simulink model "Pulse_Radar"  (R2026a)
settings: Solver=FixedStepDiscrete  StopTime=T_stop
values from neighbouring files (symbols this model uses):
  alpha = N_train * (Pfa^(-1/N_train) - 1)    (= 17.2776488339)    [init.m]
  cfar_delay = (N_train/2) + (N_guard/2)    (= 116)    [init.m]
  current_seed = randi(100000)    [init.m]    (also in run_monte_carlo.m)
  doppler_window = hamming(N_cpi)'    [init.m]
  drop_threshold_delay = 8    [init.m]
  fd = (2 * target_velocity) / lambda    [init.m]
  hardware_delay_samples = matched_filter_delay + cfar_delay + drop_threshold_delay    [init.m]
  lambda = c / fc    (= 0.03)    [init.m]
  MTI_delay = N_PRI    [init.m]
  N_cpi = 16    [init.m]
  N_delay = round(tau / Ts)    [init.m]
  N_PRI = round(PRI / Ts)    [init.m]
  N_tau_p = round(tau_p / Ts)    [init.m]
  noise_variance_IQ = Pn / 2    (= 3.99251989225e-15)    [init.m]
  radar_const = (Pt * G^2 * lambda^2) / (((4*pi)^3) * (R^4) * L)    [init.m]
  range_per_sample = (c * Ts) / 2    (= 150)    [init.m]
  sigma_avg = 1    [init.m]
  T_stop = N_cpi * PRI    (= 0.016)    [init.m]
  Ts = 1e-6    (= 1e-06)    [init.m]
  V_rx = sqrt(Pr)    [init.m]
undefined symbols (not defined in the file or in its folder): cfar_window, dspblkCoreblockFVToolHelper, gcbh, get, jet, magnitude, Radix
libraries: dspobslib x2, dspxfrm3 x1, simulink x1
settings Model: Creator=daksh  LastModifiedBy=daksh

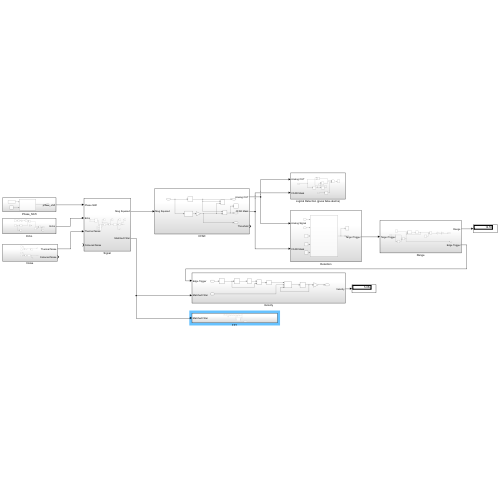
[thumbnail: Simulink's stored preview of the top-level diagram]
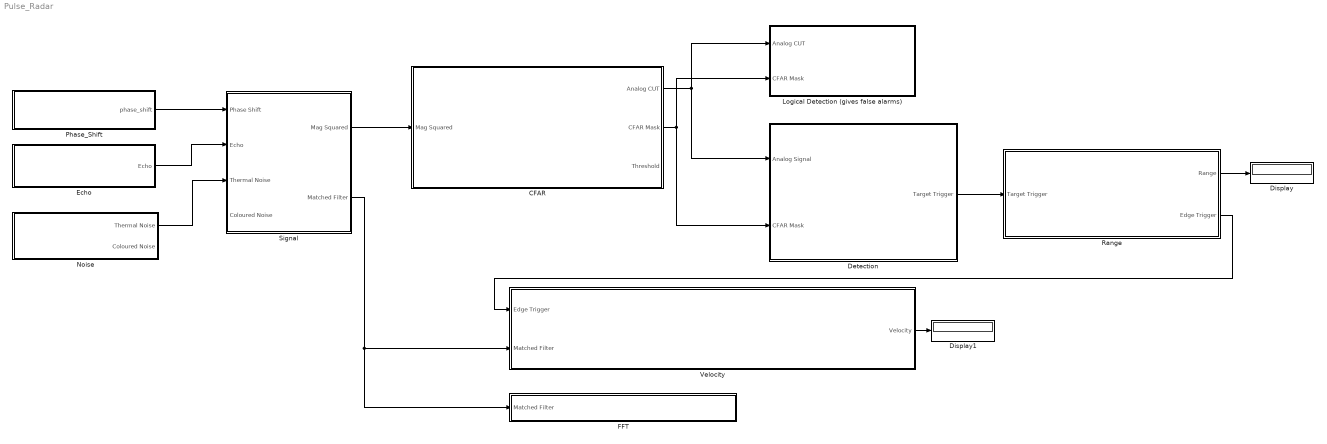
== system Pulse_Radar ==
  CFAR : Subsystem
  Detection : Subsystem
  Display : Display
  Display1 : Display
  Echo : Subsystem
  FFT : Subsystem
  Logical Detection (gives false alarms) : Subsystem
  Noise : Subsystem
  Phase_Shift : Subsystem
  Range : Subsystem
  Signal : Subsystem
  Velocity : Subsystem
  wires:
  Range/1(Range) -> Display/1
  Velocity/1(Velocity) -> Display1/1
  Echo/1(Echo) -> Signal/2(Echo)
  Noise/1(Thermal Noise) -> Signal/3(Thermal Noise)
  Signal/2(Matched Filter) -> Velocity/2(Matched Filter), FFT/1(Matched Filter)
  Signal/1(Mag Squared) -> CFAR/1(Mag Squared)
  CFAR/1(Analog CUT) -> Logical Detection (gives false alarms)/1(Analog CUT), Detection/1(Analog Signal)
  CFAR/2(CFAR Mask) -> Detection/2(CFAR Mask), Logical Detection (gives false alarms)/2(CFAR Mask)
  Detection/1(Target Trigger) -> Range/1(Target Trigger)
  Range/2(Edge Trigger) -> Velocity/1(Edge Trigger)
  Phase_Shift/1(phase_shift) -> Signal/1(Phase Shift)

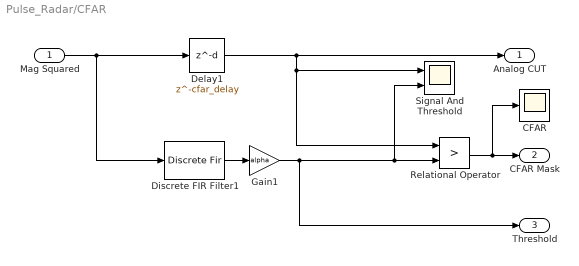
== system Pulse_Radar/CFAR ==
  Mag Squared : Inport
  CFAR : Scope
      settings: ActiveDisplayYMinimum=-0.12499999999999997  ActiveDisplayYMaximum=1.125  DataLoggingVariableName=ScopeData10
  Delay1 : Delay  DelayLength=cfar_delay
  Discrete FIR Filter1 : DiscreteFir  LoadFcn=dspblkCoreblockFVToolHelper(gcbh,'load');  Coefficients=cfar_window
      settings: CopyFcn=dspblkCoreblockFVToolHelper(gcbh,'copy');  DeleteFcn=dspblkCoreblockFVToolHelper(gcbh,'close');  ModelCloseFcn=dspblkCoreblockFVToolHelper(gcbh,'close');  PreSaveFcn=dspblkCoreblockFVToolHelper(gcbh,'presave');  PostSaveFcn=dspblkCoreblockFVToolHelper(gcbh,'postsave');  CloseFcn=dspblkCoreblockFVToolHelper(gcbh,'close');
  Gain1 : Gain  Gain=alpha
  Relational Operator : RelationalOperator  Operator=>  OutDataTypeStr=boolean  RndMeth=Simplest  InputSameDT=off
  Signal And Threshold : Scope  NumInputPorts=2
      settings: ActiveDisplayYMinimum=-1.3778826486130848E-11  ActiveDisplayYMaximum=1.2400943837517766E-10  DataLoggingVariableName=ScopeData9
  Analog CUT : Outport
  CFAR Mask : Outport  Port=2
  Threshold : Outport  Port=3
  wires:
  Gain1/1 -> Signal And Threshold/2, Relational Operator/2, Threshold/1
  Discrete FIR Filter1/1 -> Gain1/1
  Mag Squared/1 -> Discrete FIR Filter1/1, Delay1/1
  Relational Operator/1 -> CFAR/1, CFAR Mask/1
  Delay1/1 -> Relational Operator/1, Signal And Threshold/1, Analog CUT/1

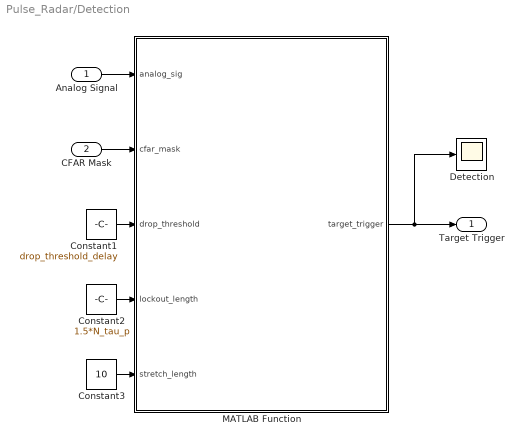
== system Pulse_Radar/Detection ==
  Analog Signal : Inport
  CFAR Mask : Inport  Port=2
  Constant1 : Constant  Value=drop_threshold_delay
  Constant2 : Constant  Value=1.5*N_tau_p
  Constant3 : Constant  Value=10
  Detection : Scope
      settings: ActiveDisplayYMinimum=-1  ActiveDisplayYMaximum=1  DataLoggingVariableName=ScopeData9
  MATLAB Function : MATLAB Function  TreatAsAtomicUnit=on
  Target Trigger : Outport
  wires:
  Constant3/1 -> MATLAB Function/5(stretch_length)
  Constant1/1 -> MATLAB Function/3(drop_threshold)
  Constant2/1 -> MATLAB Function/4(lockout_length)
  Analog Signal/1 -> MATLAB Function/1(analog_sig)
  CFAR Mask/1 -> MATLAB Function/2(cfar_mask)
  MATLAB Function/1(target_trigger) -> Detection/1, Target Trigger/1

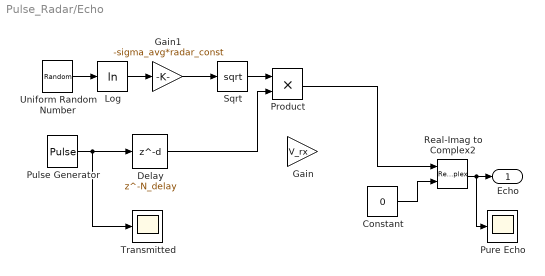
== system Pulse_Radar/Echo ==
  Constant : Constant  Value=0
  Delay : Delay  DelayLength=N_delay
  Gain : Gain  Gain=V_rx
  Gain1 : Gain  Gain=-sigma_avg*radar_const
  Log : Math  Operator=log
  Product : Product
  Pulse Generator : DiscretePulseGenerator  Period=N_PRI  PulseWidth=N_tau_p  SampleTime=Ts
  Pure Echo : Scope
      settings: ActiveDisplayYMinimum=-1.6716928323855177E-7  ActiveDisplayYMaximum=1.5045235491469661E-6  DataLoggingVariableName=ScopeData2
  Real-Imag to Complex2 : RealImagToComplex
  Sqrt : Sqrt
  Transmitted : Scope
      settings: ActiveDisplayYMinimum=-0.12499999999999997  ActiveDisplayYMaximum=1.125  DataLoggingVariableName=ScopeData3
  Uniform Random Number : UniformRandomNumber  Minimum=0.0001  Seed=current_seed  SampleTime=T_stop
  Echo : Outport
  wires:
  Pulse Generator/1 -> Transmitted/1, Delay/1
  Constant/1 -> Real-Imag to Complex2/2
  Real-Imag to Complex2/1 -> Pure Echo/1, Echo/1
  Uniform Random Number/1 -> Log/1
  Log/1 -> Gain1/1
  Gain1/1 -> Sqrt/1
  Sqrt/1 -> Product/1
  Delay/1 -> Product/2
  Product/1 -> Real-Imag to Complex2/1

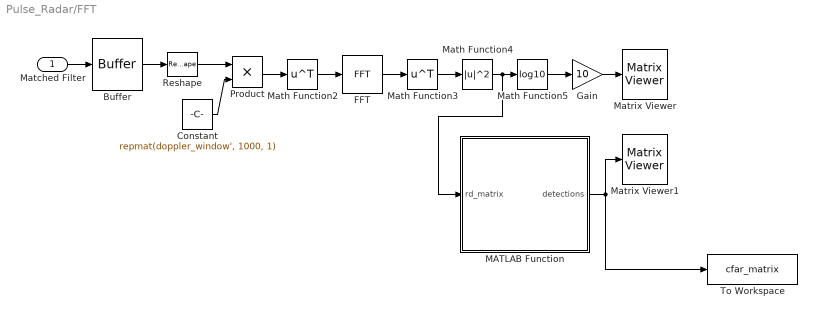
== system Pulse_Radar/FFT ==
  Matched Filter : Inport
  Buffer : Buffer  N=N_PRI*N_cpi  OutputFrames=off
  Constant : Constant  Value=repmat(doppler_window', 1000, 1)  VectorParams1D=off
  FFT : dspxfrm3/FFT  FFTImplementation=Radix-2  CompMethod=Table lookup  TableOpt=NEW  TableOptActive=Speed  BitRevOrder=off  Normalize=off  InheritFFTLength=on  FFTLength=64  WrapInput=on  roundingMode=Ceiling  overflowMode=off  firstCoeffDataTypeStr=Inherit: Same word length as input  firstCoeffLastDataTypeStr=Inherit: Same word length as input  outputMin=[]  outputMax=[]
  Gain : Gain  Gain=10
  MATLAB Function : MATLAB Function  TreatAsAtomicUnit=on
  Math Function2 : Math  Operator=transpose
  Math Function3 : Math  Operator=transpose
  Math Function4 : Math  Operator=magnitude^2
  Math Function5 : Math  Operator=log10
  Matrix Viewer : dspobslib/Matrix Viewer  ImageParams=off  CMapStr=jet(256)  AxisColorbar=on  AxisParams=off  AxisOrigin=Upper left corner  AxisTickMode=Auto  XTickRange=[0 1]  YTickRange=[0 1]  XLabel=X-axis  YLabel=Y-axis  ZLabel=Z-axis  FigPos=get(0,'defaultfigureposition')  AxisZoom=off
      settings: YMin=-100  YMax=0
  Matrix Viewer1 : dspobslib/Matrix Viewer  ImageParams=off  CMapStr=gray  AxisColorbar=on  AxisParams=off  AxisOrigin=Upper left corner  AxisTickMode=Auto  XTickRange=[0 1]  YTickRange=[0 1]  XLabel=X-axis  YLabel=Y-axis  ZLabel=Z-axis  FigPos=get(0,'defaultfigureposition')  AxisZoom=off
      settings: YMin=0  YMax=1
  Product : Product
  Reshape : Reshape  OutputDimensionality=Customize  OutputDimensions=[N_PRI, N_cpi]
  To Workspace : ToWorkspace  VariableName=cfar_matrix  SampleTime=-1
  wires:
  Math Function5/1 -> Gain/1
  Math Function3/1 -> Math Function4/1
  FFT/1 -> Math Function3/1
  Gain/1 -> Matrix Viewer/1
  Math Function4/1 -> MATLAB Function/1(rd_matrix), Math Function5/1
  Math Function2/1 -> FFT/1
  Buffer/1 -> Reshape/1
  Matched Filter/1 -> Buffer/1
  MATLAB Function/1(detections) -> Matrix Viewer1/1, To Workspace/1
  Reshape/1 -> Product/1
  Constant/1 -> Product/2
  Product/1 -> Math Function2/1

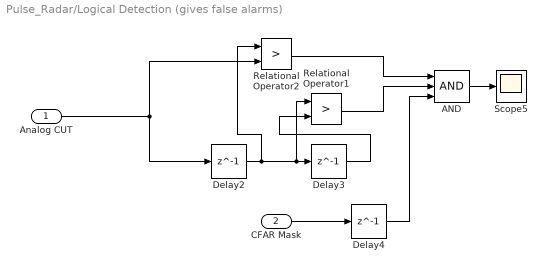
== system Pulse_Radar/Logical Detection (gives false alarms) ==
  Analog CUT : Inport
  CFAR Mask : Inport  Port=2
  AND : Logic  Inputs=3  IconShape=distinctive  AllPortsSameDT=off  OutDataTypeStr=boolean
  Delay2 : Delay  DelayLength=1
  Delay3 : Delay  DelayLength=1
  Delay4 : Delay  DelayLength=1
  Relational Operator1 : RelationalOperator  Operator=>  OutDataTypeStr=boolean  RndMeth=Simplest  InputSameDT=off
  Relational Operator2 : RelationalOperator  Operator=>  OutDataTypeStr=boolean  RndMeth=Simplest  InputSameDT=off
  Scope5 : Scope
      settings: ActiveDisplayYMinimum=-0.12499999999999997  ActiveDisplayYMaximum=1.125  DataLoggingVariableName=ScopeData5
  wires:
  Relational Operator2/1 -> AND/1
  AND/1 -> Scope5/1
  Delay2/1 -> Relational Operator2/1, Relational Operator1/1, Delay3/1
  Delay3/1 -> Relational Operator1/2
  Relational Operator1/1 -> AND/2
  Delay4/1 -> AND/3
  Analog CUT/1 -> Delay2/1, Relational Operator2/2
  CFAR Mask/1 -> Delay4/1

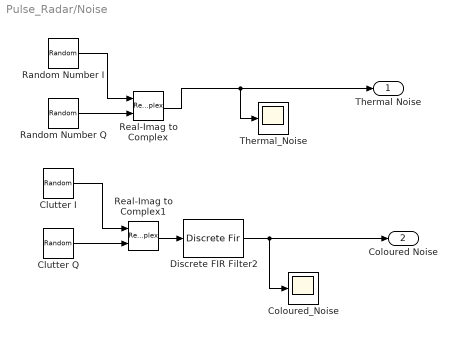
== system Pulse_Radar/Noise ==
  Clutter I : RandomNumber  Variance=noise_variance_IQ*50  Seed=69  SampleTime=Ts
  Clutter Q : RandomNumber  Variance=noise_variance_IQ*50  Seed=67  SampleTime=Ts
  Coloured_Noise : Scope
      settings: ActiveDisplayYMinimum=-1  ActiveDisplayYMaximum=1
  Discrete FIR Filter2 : DiscreteFir  LoadFcn=dspblkCoreblockFVToolHelper(gcbh,'load');  Coefficients=ones(1,100)/10
      settings: CopyFcn=dspblkCoreblockFVToolHelper(gcbh,'copy');  DeleteFcn=dspblkCoreblockFVToolHelper(gcbh,'close');  ModelCloseFcn=dspblkCoreblockFVToolHelper(gcbh,'close');  PreSaveFcn=dspblkCoreblockFVToolHelper(gcbh,'presave');  PostSaveFcn=dspblkCoreblockFVToolHelper(gcbh,'postsave');  CloseFcn=dspblkCoreblockFVToolHelper(gcbh,'close');
  Random Number I : RandomNumber  Variance=noise_variance_IQ  SampleTime=Ts
  Random Number Q : RandomNumber  Variance=noise_variance_IQ  Seed=123  SampleTime=Ts
  Real-Imag to Complex : RealImagToComplex
  Real-Imag to Complex1 : RealImagToComplex
  Thermal_Noise : Scope
      settings: ActiveDisplayYMinimum=-3.1205725347729866E-7  ActiveDisplayYMaximum=3.0716380696194773E-7
  Thermal Noise : Outport
  Coloured Noise : Outport  Port=2
  wires:
  Real-Imag to Complex/1 -> Thermal_Noise/1, Thermal Noise/1
  Random Number I/1 -> Real-Imag to Complex/1
  Random Number Q/1 -> Real-Imag to Complex/2
  Clutter I/1 -> Real-Imag to Complex1/1
  Clutter Q/1 -> Real-Imag to Complex1/2
  Real-Imag to Complex1/1 -> Discrete FIR Filter2/1
  Discrete FIR Filter2/1 -> Coloured_Noise/1, Coloured Noise/1

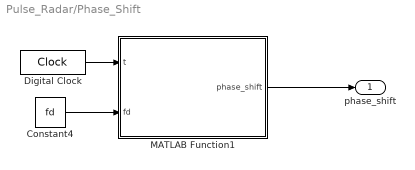
== system Pulse_Radar/Phase_Shift ==
  Constant4 : Constant  Value=fd
  Digital Clock : DigitalClock  SampleTime=Ts
  MATLAB Function1 : MATLAB Function  TreatAsAtomicUnit=on
  phase_shift : Outport
  wires:
  Digital Clock/1 -> MATLAB Function1/1(t)
  Constant4/1 -> MATLAB Function1/2(fd)
  MATLAB Function1/1(phase_shift) -> phase_shift/1

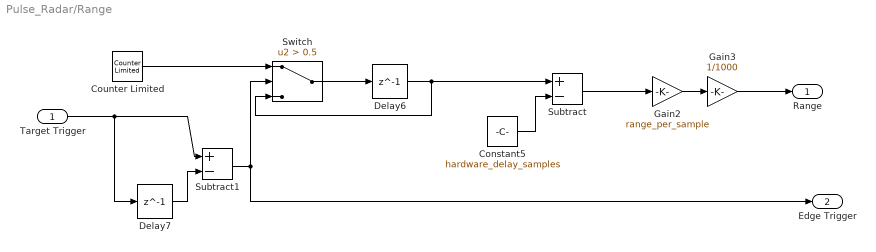
== system Pulse_Radar/Range ==
  Target Trigger : Inport
  Constant5 : Constant  Value=hardware_delay_samples
  Counter Limited : simulink/Sources/Counter Limited  uplimit=N_PRI-1  tsamp=Ts
  Delay6 : Delay  DelayLength=1
  Delay7 : Delay  DelayLength=1
  Gain2 : Gain  Gain=range_per_sample
  Gain3 : Gain  Gain=1/1000
  Subtract : Sum  Inputs=+-
  Subtract1 : Sum  Inputs=+-
  Switch : Switch  Criteria=u2 > Threshold  Threshold=0.5  SaturateOnIntegerOverflow=off  InputSameDT=off
  Range : Outport
  Edge Trigger : Outport  Port=2
  wires:
  Subtract1/1 -> Edge Trigger/1, Switch/2
  Delay7/1 -> Subtract1/2
  Subtract/1 -> Gain2/1
  Constant5/1 -> Subtract/2
  Delay6/1 -> Subtract/1, Switch/3
  Switch/1 -> Delay6/1
  Counter Limited/1 -> Switch/1
  Gain2/1 -> Gain3/1
  Target Trigger/1 -> Delay7/1, Subtract1/1
  Gain3/1 -> Range/1

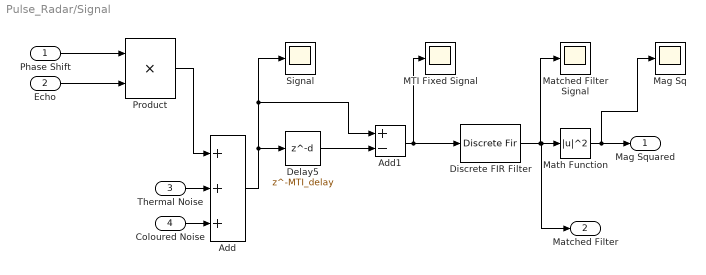
== system Pulse_Radar/Signal ==
  Phase Shift : Inport
  Echo : Inport  Port=2
  Thermal Noise : Inport  Port=3
  Coloured Noise : Inport  Port=4
  Add : Sum  Inputs=+++
  Add1 : Sum  Inputs=+-
  Delay5 : Delay  DelayLength=MTI_delay
  Discrete FIR Filter : DiscreteFir  LoadFcn=dspblkCoreblockFVToolHelper(gcbh,'load');  Coefficients=range_window'
      settings: CopyFcn=dspblkCoreblockFVToolHelper(gcbh,'copy');  DeleteFcn=dspblkCoreblockFVToolHelper(gcbh,'close');  ModelCloseFcn=dspblkCoreblockFVToolHelper(gcbh,'close');  PreSaveFcn=dspblkCoreblockFVToolHelper(gcbh,'presave');  PostSaveFcn=dspblkCoreblockFVToolHelper(gcbh,'postsave');  CloseFcn=dspblkCoreblockFVToolHelper(gcbh,'close');
  MTI Fixed Signal : Scope
      settings: ActiveDisplayYMinimum=-3.2187633765663632E-6  ActiveDisplayYMaximum=3.1799471834312863E-6  DataLoggingVariableName=ScopeData6
  Mag Sq : Scope
      settings: ActiveDisplayYMinimum=-4.0400443525082573E-10  ActiveDisplayYMaximum=3.6360438986890831E-9  DataLoggingVariableName=ScopeData8
  Matched Filter Signal : Scope
      settings: ActiveDisplayYMinimum=-6.9752281906762913E-5  ActiveDisplayYMaximum=7.01926675670559E-5  DataLoggingVariableName=ScopeData7
  Math Function : Math  Operator=magnitude^2
  Product : Product
  Signal : Scope
      settings: ActiveDisplayYMinimum=-1.8860280451870471E-6  ActiveDisplayYMaximum=1.9010273466324376E-6  DataLoggingVariableName=ScopeData4
  Mag Squared : Outport
  Matched Filter : Outport  Port=2
  wires:
  Add1/1 -> MTI Fixed Signal/1, Discrete FIR Filter/1
  Delay5/1 -> Add1/2
  Product/1 -> Add/1
  Add/1 -> Signal/1, Add1/1, Delay5/1
  Thermal Noise/1 -> Add/2
  Coloured Noise/1 -> Add/3
  Math Function/1 -> Mag Sq/1, Mag Squared/1
  Discrete FIR Filter/1 -> Matched Filter Signal/1, Matched Filter/1, Math Function/1
  Phase Shift/1 -> Product/1
  Echo/1 -> Product/2

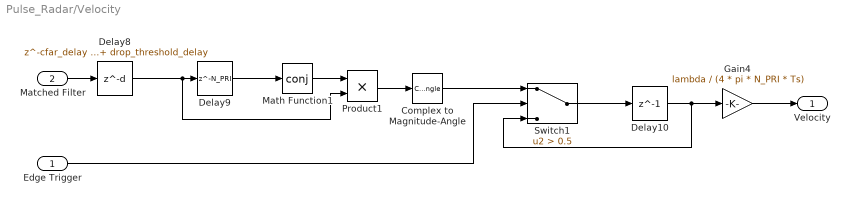
== system Pulse_Radar/Velocity ==
  Edge Trigger : Inport
  Matched Filter : Inport  Port=2
  Complex to Magnitude-Angle : ComplexToMagnitudeAngle  Output=Angle
  Delay10 : Delay  DelayLength=1
  Delay8 : Delay  DelayLength=cfar_delay + drop_threshold_delay
  Delay9 : Delay  DelayLength=N_PRI
  Gain4 : Gain  Gain=lambda / (4 * pi * N_PRI * Ts)
  Math Function1 : Math  Operator=conj
  Product1 : Product
  Switch1 : Switch  Criteria=u2 > Threshold  Threshold=0.5  SaturateOnIntegerOverflow=off  InputSameDT=off
  Velocity : Outport
  wires:
  Delay9/1 -> Math Function1/1
  Delay10/1 -> Gain4/1, Switch1/3
  Delay8/1 -> Product1/2, Delay9/1
  Product1/1 -> Complex to Magnitude-Angle/1
  Complex to Magnitude-Angle/1 -> Switch1/1
  Math Function1/1 -> Product1/1
  Switch1/1 -> Delay10/1
  Matched Filter/1 -> Delay8/1
  Gain4/1 -> Velocity/1
  Edge Trigger/1 -> Switch1/2

== matlab function Pulse_Radar/Phase_Shift/MATLAB Function1 ==
  data: t input; phase_shift output; fd input
function phase_shift = apply_doppler(t, fd)
    phase_shift = exp(1j * 2 * pi * fd * t);
end

== matlab function Pulse_Radar/FFT/MATLAB Function ==
  data: rd_matrix input; detections output
function detections = cfar_2d(rd_matrix)
    % rd_matrix must be 1000x16 Linear Power (|u|^2)
    [num_ranges, num_dopplers] = size(rd_matrix);
% --- 2D CFAR Parameters ---
    Pfa = 1e-6;     % Probability of False Alarm
    Tr = 16;        % Training cells in Range (Vertical)
    Td = 1;         % Training cells in Doppler (Horizontal)
    
    Gr = 100;       % Guard cells in Range (clears the 200-sample triangle)
    Gd = 1;         % FIX: Guard cells in Doppler (clears FFT leakage)
    
    % Calculate the number of training cells in the 2D "donut"
    N_train = (2*(Tr+Gr)+1)*(2*(Td+Gd)+1) - (2*Gr+1)*(2*Gd+1);
    
    % Threshold Multiplier (alpha)
    alpha = N_train * (Pfa^(-1/N_train) - 1);
    
    % Preallocate the output binary map
    detections = zeros(num_ranges, num_dopplers);
    
    % --- The Sliding 2D Window ---
    % We loop only through the "valid" center of the matrix to avoid edge crashes
    for r = (Tr+Gr+1) : (num_ranges - (Tr+Gr))
        for d = (Td+Gd+1) : (num_dopplers - (Td+Gd))
            
            % 1. Extract the entire outer window
            window = rd_matrix(r-(Tr+Gr) : r+(Tr+Gr), d-(Td+Gd) : d+(Td+Gd));
            
            % 2. Extract the inner guard region (including CUT)
            guard = rd_matrix(r-Gr : r+Gr, d-Gd : d+Gd);
            
            % 3. Calculate the noise average (Outer Window - Inner Guard)
            noise_sum = sum(window(:)) - sum(guard(:));
            noise_avg = noise_sum / N_train;
            
            % 4. Apply threshold to the Cell Under Test (CUT)
            threshold = noise_avg * alpha;
            cut = rd_matrix(r, d);
            
            % 5. Declare Detection
            if cut > threshold
                detections(r, d) = 1;
            end
        end
    end
end

== matlab function Pulse_Radar/Detection/MATLAB Function ==
  data: analog_sig input; target_trigger output; cfar_mask input; drop_threshold input; lockout_length input; stretch_length input
function target_trigger = extract_plot(analog_sig, cfar_mask, drop_threshold, lockout_length, stretch_length)
    % persistent memory registers
    persistent drop_counter lockout_timer last_sig display_timer;
    
    if isempty(drop_counter)
        drop_counter = 0;
        lockout_timer = 0;
        last_sig = 0;
        display_timer = 0;
    end
    
    target_trigger = 0;
    
    % 1. Scope Stretcher (Visual)
    if display_timer > 0
        target_trigger = 1;
        display_timer = display_timer - 1;
    end
    
    % 2. Advance Lockout
    if lockout_timer > 0
        lockout_timer = lockout_timer - 1;
    end
    
    % 3. Peak Detection Logic
    if cfar_mask == 1 && lockout_timer == 0
        
        if analog_sig < last_sig
            drop_counter = drop_counter + 1;
        else
            drop_counter = 0; % Reset on any rise
        end
        
        % The hardcoded 5 is now dynamically controlled by drop_threshold
        if drop_counter == drop_threshold
            target_trigger = 1;      
            display_timer = stretch_length;      
            lockout_timer = lockout_length;     
            drop_counter = 0;        
        end
        
    else
        drop_counter = 0;
    end
    
    last_sig = analog_sig;
end
